simulink model "Non_linear_simulation"  (R2020b)
settings: Solver=ode45  StartTime=0.0  StopTime=10  FixedStep=.002  RelTol=1e-3  EnableMultiTasking=on
undefined symbols (not defined in the file): alphaPlotHandle, armPartPatchHandle, armPartVertices, Bp, Br, drivePartPatchHandle, drivePartVertices, eta_g, eta_m, frameRate, G, g, J, Jp, kb, kt, Lp, lp, mp, pendPartPatchHandle, pendPartVertices, r, Ra, thetaPlotHandle
settings Model: Creator=Dylan  LastModifiedBy=dcanb
settings SolverCC: DecoupledContinuousIntegration=on
settings DataIOCC: LimitDataPoints=on  SaveFormat=StructureWithTime  ReturnWorkspaceOutputs=off
settings OptimizationCC: LifeSpan=inf
settings DebuggingCC: AllowSymbolicDim=off  SFUnexpectedBacktrackingDiag=warning  SFNoUnconditionalDefaultTransitionDiag=warning  SFExecutionAtInitializationDiag=none  ArithmeticOperatorsInVariantConditions=warning
settings HardwareCC: ProdBitPerSizeT=32  ProdBitPerPtrDiffT=32  ProdWordSize=32  ProdHWDeviceType=Specified
settings ModelReferenceCC: PropagateSignalLabelsOutOfModel=off
settings SFSimCC: SimUseLocalCustomCode=off  CustomCodeUndefinedFunction=UseInterfaceOnly  SimTargetLang=C++  GPUAcceleration=on  SimDLTargetLibrary=cudnn
settings RTWCC: RTWUseLocalCustomCode=off
settings CodeAppCC: StateflowObjectComments=on
settings GRTTargetCC: TargetLangStandard=C89/C90 (ANSI)
settings ConfigComp: CovMetricSettings=dw  CovSaveCumulativeToWorkspaceVar=on  CovSaveSingleToWorkspaceVar=on  CovExternalEMLEnable=off

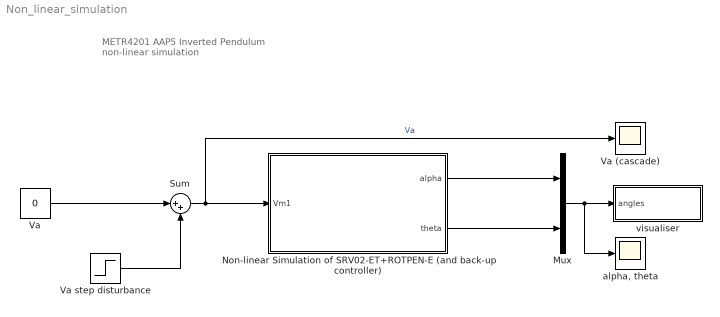
== system Non_linear_simulation ==
  note: METR4201 AAP5
      | Inverted Pendulum non-linear simulation
  Mux : Mux  Inputs=2
  Non-linear Simulation of SRV02-ET+ROTPEN-E (and back-up controller) : Subsystem
  Sum : Sum  Inputs=|++
  Va : Constant  Value=0
  Va (cascade) : Scope
  Va step disturbance : Step  SampleTime=0
  "alpha, theta" : Scope
  visualiser : Subsystem
  wires:
  Mux/1 -> "alpha, theta"/1, visualiser/1(angles)
  Non-linear Simulation of SRV02-ET+ROTPEN-E (and back-up controller)/2(theta) -> Mux/2
  Non-linear Simulation of SRV02-ET+ROTPEN-E (and back-up controller)/1(alpha) -> Mux/1
  Sum/1 -> Va (cascade)/1, Non-linear Simulation of SRV02-ET+ROTPEN-E (and back-up controller)/1(Vm1)  "Va"
  Va step disturbance/1 -> Sum/2
  Va/1 -> Sum/1

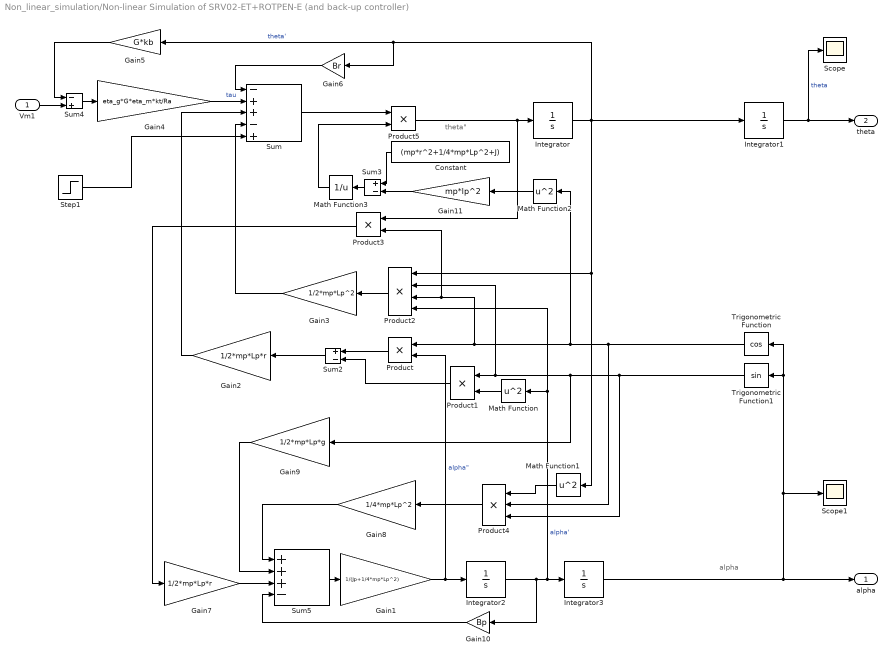
== system Non_linear_simulation/Non-linear Simulation of SRV02-ET+ROTPEN-E (and back-up controller) ==
  note: theta"
  note: alpha
  Vm1 : Inport
  Constant : Constant  Value=(mp*r^2+1/4*mp*Lp^2+J)
  Gain1 : Gain  Gain=1/(Jp+1/4*mp*Lp^2)
  Gain10 : Gain  Gain=Bp
  Gain11 : Gain  Gain=mp*lp^2
  Gain2 : Gain  Gain=1/2*mp*Lp*r
  Gain3 : Gain  Gain=1/2*mp*Lp^2
  Gain4 : Gain  Gain=eta_g*G*eta_m*kt/Ra
  Gain5 : Gain  Gain=G*kb
  Gain6 : Gain  Gain=Br
  Gain7 : Gain  Gain=1/2*mp*Lp*r
  Gain8 : Gain  Gain=1/4*mp*Lp^2
  Gain9 : Gain  Gain=1/2*mp*Lp*g
  Integrator{,1..3} (4 alike) : Integrator
  Math Function : Math  Operator=square  SignedPower=on  SaturateOnIntegerOverflow=on
  Math Function1 : Math  Operator=square  SignedPower=on  SaturateOnIntegerOverflow=on
  Math Function2 : Math  Operator=square  SignedPower=on  SaturateOnIntegerOverflow=on
  Math Function3 : Math  Operator=reciprocal  SignedPower=on  SaturateOnIntegerOverflow=on
  Product{,1,3,5} (4 alike) : Product  RndMeth=Zero
  Product2 : Product  Inputs=4  RndMeth=Zero
  Product4 : Product  Inputs=3  RndMeth=Zero
  Scope : Scope
  Scope1 : Scope
  Step1 : Step  Time=.1  After=0  SampleTime=0
  Sum : Sum  Inputs=-++-+
  Sum2 : Sum  Inputs=+-
  Sum3 : Sum  Inputs=+-
  Sum4 : Sum  Inputs=-+
  Sum5 : Sum  Inputs=+++-
  Trigonometric Function : Trigonometry  Operator=cos
  Trigonometric Function1 : Trigonometry
  alpha : Outport  VectorParamsAs1DForOutWhenUnconnected=off
  theta : Outport  Port=2  VectorParamsAs1DForOutWhenUnconnected=off
  wires:
  Product5/1 -> Product3/1, Integrator/1
  Product/1 -> Sum2/1
  Sum2/1 -> Gain2/1
  Sum/1 -> Product5/1
  Gain9/1 -> Sum5/2
  Gain10/1 -> Sum5/4
  Math Function2/1 -> Gain11/1
  Gain11/1 -> Sum3/2
  Constant/1 -> Sum3/1
  Sum3/1 -> Math Function3/1
  Math Function3/1 -> Product5/2
  Sum5/1 -> Gain1/1
  Gain2/1 -> Sum/3
  Gain7/1 -> Sum5/3
  Product3/1 -> Gain7/1
  Trigonometric Function1/1 -> Product4/3, Gain9/1, Product2/2, Product1/1
  Math Function/1 -> Product1/2
  Product1/1 -> Sum2/2
  Product4/1 -> Gain8/1
  Product2/1 -> Gain3/1
  Vm1/1 -> Sum4/2
  Gain5/1 -> Sum4/1
  Sum4/1 -> Gain4/1
  Gain4/1 -> Sum/2  "tau"
  Gain6/1 -> Sum/1
  Gain3/1 -> Sum/4
  Gain8/1 -> Sum5/1
  Math Function1/1 -> Product4/1
  Integrator2/1 -> Gain10/1, Integrator3/1, Math Function/1, Product2/4  "alpha'"
  Gain1/1 -> Product/2, Integrator2/1  "alpha\""
  Trigonometric Function/1 -> Product4/2, Product3/2, Product2/3, Product/1, Math Function2/1
  Integrator/1 -> Math Function1/1, Product2/1, Integrator1/1, Gain6/1, Gain5/1  "theta'"
  Integrator1/1 -> theta/1, Scope/1  "theta"
  Step1/1 -> Sum/5
  Integrator3/1 -> Scope1/1, Trigonometric Function/1, Trigonometric Function1/1, alpha/1

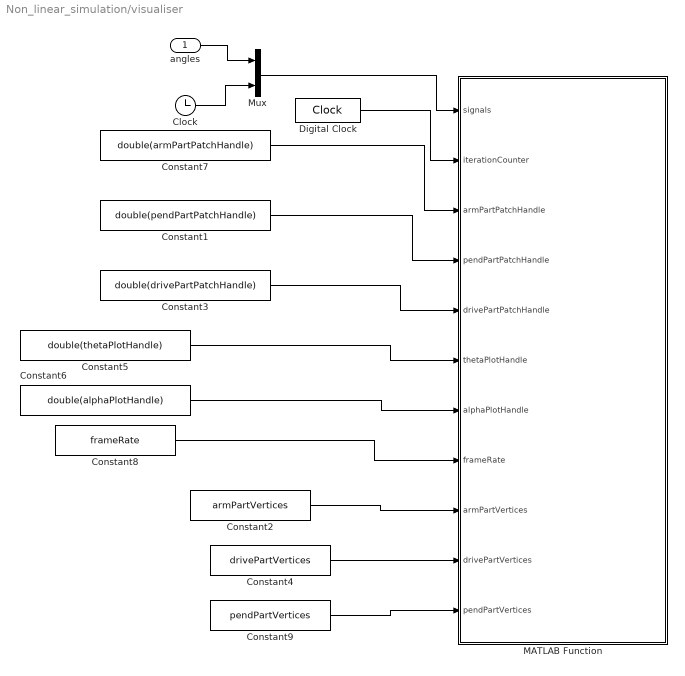
== system Non_linear_simulation/visualiser ==
  angles : Inport
  Clock : Clock
  Constant1 : Constant  Value=double(pendPartPatchHandle)
  Constant2 : Constant  Value=armPartVertices  VectorParams1D=off
  Constant3 : Constant  Value=double(drivePartPatchHandle)
  Constant4 : Constant  Value=drivePartVertices  VectorParams1D=off
  Constant5 : Constant  Value=double(thetaPlotHandle)
  Constant6 : Constant  Value=double(alphaPlotHandle)
  Constant7 : Constant  Value=double(armPartPatchHandle)
  Constant8 : Constant  Value=frameRate  VectorParams1D=off
  Constant9 : Constant  Value=pendPartVertices  VectorParams1D=off
  Digital Clock : DigitalClock  SampleTime=.001
  MATLAB Function : MATLAB Function  TreatAsAtomicUnit=on
  Mux : Mux  Inputs=2
  wires:
  angles/1 -> Mux/1
  Mux/1 -> MATLAB Function/1(signals)
  Clock/1 -> Mux/2
  Constant7/1 -> MATLAB Function/3(armPartPatchHandle)
  Constant1/1 -> MATLAB Function/4(pendPartPatchHandle)
  Constant6/1 -> MATLAB Function/7(alphaPlotHandle)
  Constant5/1 -> MATLAB Function/6(thetaPlotHandle)
  Constant3/1 -> MATLAB Function/5(drivePartPatchHandle)
  Digital Clock/1 -> MATLAB Function/2(iterationCounter)
  Constant8/1 -> MATLAB Function/8(frameRate)
  Constant2/1 -> MATLAB Function/9(armPartVertices)
  Constant4/1 -> MATLAB Function/10(drivePartVertices)
  Constant9/1 -> MATLAB Function/11(pendPartVertices)

== matlab function Non_linear_simulation/visualiser/MATLAB Function ==
  data: signals input; iterationCounter input; armPartPatchHandle input; pendPartPatchHandle input; drivePartPatchHandle input; thetaPlotHandle input; alphaPlotHandle input; frameRate input; armPartVertices input; drivePartVertices input; pendPartVertices input
function  updateVisualiser(signals, iterationCounter, armPartPatchHandle, pendPartPatchHandle, drivePartPatchHandle, thetaPlotHandle, alphaPlotHandle, frameRate, armPartVertices,drivePartVertices,pendPartVertices)

%
% We need the set and get functions for changing plots.
%
coder.extrinsic('set');
coder.extrinsic('get');


%
% Clear the theta and alpha plots if this is the first iteration.
%
if iterationCounter == 0
    set(thetaPlotHandle,'xData',inf,'yData',inf);
    set(alphaPlotHandle,'xData',inf,'yData',inf);
end

%
% Only update figure on every 2nd iteration.
%
if mod(iterationCounter,1/frameRate) == 0
    
    alphaAngle = signals(1);
    thetaAngle = signals(2);
    currentTime = signals(3);
    
    %
    % New frame transformations.
    %
    BaseToArm = homogeneous_func(0,0,thetaAngle,0,0,12e-2);
    ArmToPendulum = homogeneous_func(alphaAngle,0,0,14.2e-2,0,5e-2);
    BaseToDrive = homogeneous_func(0,0,(-thetaAngle*5),0,0.036,12e-2);
    
    %
    % Update arm parts.
    %
    armPart_vertices_G_frame = BaseToArm * armPartVertices;
    Xt = reshape(armPart_vertices_G_frame(1,:),3,[]);
    Yt = reshape(armPart_vertices_G_frame(2,:),3,[]);
    Zt = reshape(armPart_vertices_G_frame(3,:),3,[]);
    set(armPartPatchHandle, 'xData', Xt, 'yData', Yt, 'zData', Zt);
    
    %
    % Update pendulum parts.
    %
    pendPart_vertices_G_frame = BaseToArm * ArmToPendulum* pendPartVertices;
    Xt = reshape(pendPart_vertices_G_frame(1,:),3,[]);
    Yt = reshape(pendPart_vertices_G_frame(2,:),3,[]);
    Zt = reshape(pendPart_vertices_G_frame(3,:),3,[]);
    set(pendPartPatchHandle, 'xData', Xt, 'yData', Yt, 'zData', Zt);
    
    %
    % Update drive gear parts.
    %
    drivePart_vertices_G_frame = BaseToDrive* drivePartVertices;
    Xt = reshape(drivePart_vertices_G_frame(1,:),3,[]);
    Yt = reshape(drivePart_vertices_G_frame(2,:),3,[]);
    Zt = reshape(drivePart_vertices_G_frame(3,:),3,[]);
    set(drivePartPatchHandle, 'xData', Xt, 'yData', Yt, 'zData', Zt);
    
    %
    % Update theta plot.
    %
    times = [get(thetaPlotHandle,'xData'), currentTime];
    thetaAngles = [get(thetaPlotHandle,'yData'), thetaAngle*180/pi];
    set(thetaPlotHandle,'xdata',times,'ydata',thetaAngles);
    
    %
    % Update alpha plot.
    %
    times = [get(alphaPlotHandle,'xData'), currentTime];
    alphaAngles = [get(alphaPlotHandle,'yData'), alphaAngle*180/pi];
    set(alphaPlotHandle,'xdata',times,'ydata',alphaAngles);
end
end

function [T] = homogeneous_func(ROLL, PITCH, YAW, X, Y, Z)
cy=cos(YAW);
cp=cos(PITCH);
cr=cos(ROLL);
sp=sin(PITCH);
sr=sin(ROLL);
sy=sin(YAW);
T=[cy*cp, cy*sp*sr-sy*cr, cy*sp*cr+sy*sr, X; sy*cp, sy*sp*sr+cy*cr, sy*sp*cr-cy*sr, Y;
    -sp, cp*sr, cp*cr, Z; 0,0,0,1];
end
